simulink model "Assignment1_NafizImtiaz"  (R2020b)
settings: Solver=VariableStepAuto  StartTime=0.0  StopTime=10.0  RelTol=1e-3
settings Model: Creator=derek  LastModifiedBy=hp

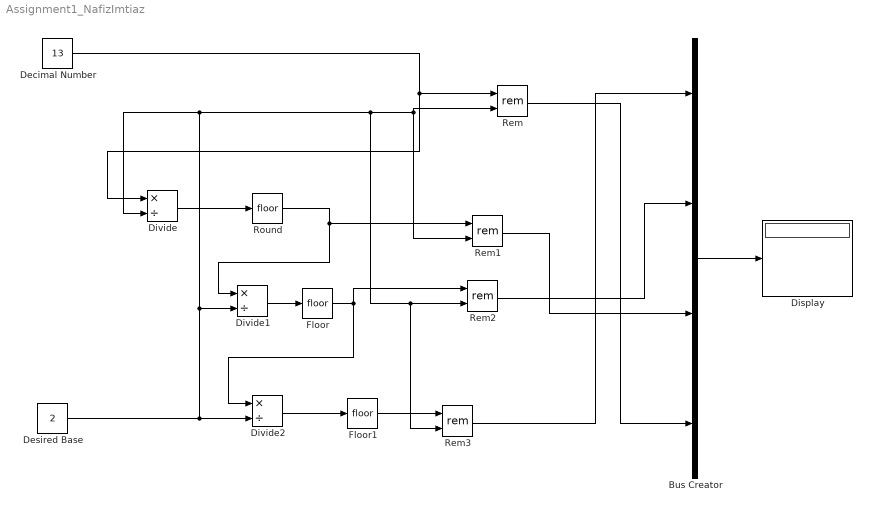
== system Assignment1_NafizImtiaz ==
  Bus Creator : BusCreator  Inputs=4
  Decimal Number : Constant  Value=13
  Desired Base : Constant  Value=2
  Display : Display
  Divide : Product  Inputs=*/
  Divide1 : Product  Inputs=*/
  Divide2 : Product  Inputs=*/
  Floor : Rounding
  Floor1 : Rounding
  Rem{,1..3} (4 alike) : Math  Operator=rem  SaturateOnIntegerOverflow=on
  Round : Rounding
  wires:
  Bus Creator/1 -> Display/1
  Decimal Number/1 -> Divide/1, Rem/1
  Desired Base/1 -> Rem3/2, Rem2/2, Rem1/2, Rem/2, Divide/2, Divide1/2, Divide2/2
  Divide/1 -> Round/1
  Round/1 -> Divide1/1, Rem1/1
  Divide1/1 -> Floor/1
  Floor/1 -> Divide2/1, Rem2/1
  Divide2/1 -> Floor1/1
  Floor1/1 -> Rem3/1
  Rem3/1 -> Bus Creator/1
  Rem2/1 -> Bus Creator/2
  Rem1/1 -> Bus Creator/3
  Rem/1 -> Bus Creator/4
